simulink model "debugIMU"  (Simulink 9.0)
settings: Solver=FixedStepDiscrete  StartTime=0.0  StopTime=inf  FixedStep=0.01  RelTol=1e-3  EnableMultiTasking=on
InitFcn:
  | ROBOT_DOF=23;
libraries: WBToolboxLibrary x6
settings Model: SuppressorTable=22 serialization::archive 11 0 6 0 0 0 11 0  Creator=DanielePucci  LastModifiedBy=icub
settings DataIOCC: LimitDataPoints=on  SaveFormat=StructureWithTime
settings DebuggingCC: UnderspecifiedInitializationDetection=Simplified  MergeDetectMultiDrivingBlocksExec=error
settings HardwareCC: ProdBitPerPointer=64  ProdLargestAtomicFloat=Float  ProdIntDivRoundTo=Zero  ProdEndianess=LittleEndian  ProdHWDeviceType=Specified

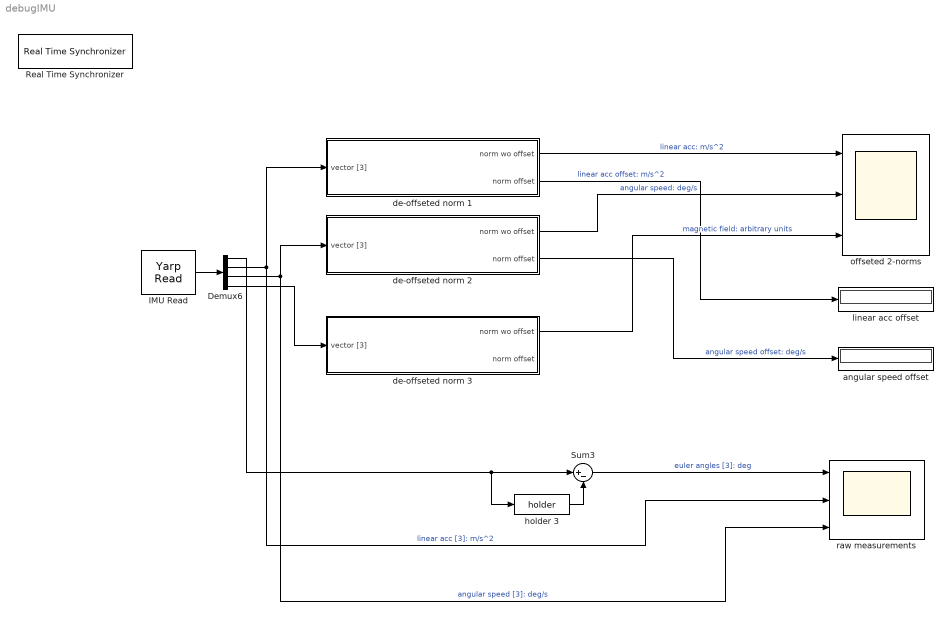
== system debugIMU ==
  Demux6 : Demux
  IMU Read : WBToolboxLibrary/Utilities/Yarp Read  portName='/icub/inertial'  signalSize=12  blocking=off  timestamp=off  autoconnect=on  errorOnConnection=off
      settings: SourceProductName=Whole Body Toolbox
  Real Time Synchronizer : WBToolboxLibrary/Utilities/Real Time Synchronizer  period=0.01
      settings: SourceProductName=Whole Body Toolbox
  Sum3 : Sum  Inputs=|+-
  angular speed offset : Display
  de-offseted norm 1 : Subsystem
  de-offseted norm 2 : Subsystem
  de-offseted norm 3 : Subsystem
  holder 3 : WBToolboxLibrary/Utilities/holder 
      settings: SourceProductName=Whole Body Toolbox
  linear acc offset : Display
  offseted 2-norms : Scope  NumInputPorts=3
  raw measurements : Scope  NumInputPorts=3
  wires:
  IMU Read/1 -> Demux6/1
  de-offseted norm 2/2(norm offset) -> angular speed offset/1  "angular speed offset: deg/s"
  de-offseted norm 2/1(norm wo offset) -> offseted 2-norms/2  "angular speed: deg/s"
  de-offseted norm 3/1(norm wo offset) -> offseted 2-norms/3  "magnetic field: arbitrary units"
  Demux6/2 -> de-offseted norm 1/1(vector [3]), raw measurements/2  "linear acc [3]: m/s^2"
  Demux6/3 -> de-offseted norm 2/1(vector [3]), raw measurements/3  "angular speed [3]: deg/s"
  Demux6/4 -> de-offseted norm 3/1(vector [3])
  Sum3/1 -> raw measurements/1  "euler angles [3]: deg"
  Demux6/1 -> holder 3/1, Sum3/1
  holder 3/1 -> Sum3/2
  de-offseted norm 1/1(norm wo offset) -> offseted 2-norms/1  "linear acc: m/s^2"
  de-offseted norm 1/2(norm offset) -> linear acc offset/1  "linear acc offset: m/s^2"

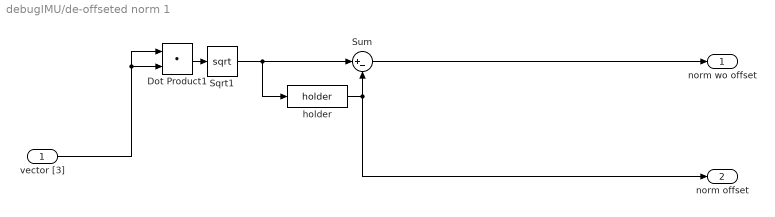
== system debugIMU/de-offseted norm 1 ==
  vector [3] : Inport
  Dot Product1 : DotProduct  InputSameDT=on  OutDataTypeStr=Inherit: Inherit via internal rule
  Sqrt1 : Sqrt  SaturateOnIntegerOverflow=on
  Sum : Sum  Inputs=|+-
  "holder " : WBToolboxLibrary/Utilities/holder 
      settings: SourceProductName=Whole Body Toolbox
  norm wo offset : Outport
  norm offset : Outport  Port=2
  wires:
  "holder "/1 -> norm offset/1, Sum/2
  Sqrt1/1 -> "holder "/1, Sum/1
  Sum/1 -> norm wo offset/1
  Dot Product1/1 -> Sqrt1/1
  vector [3]/1 -> Dot Product1/1, Dot Product1/2

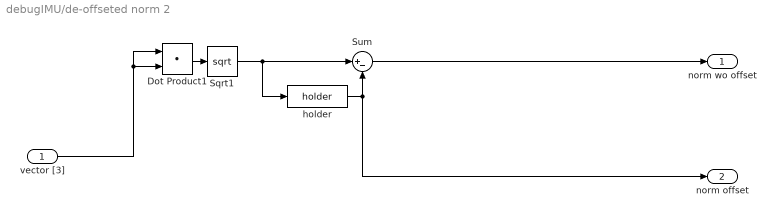
== system debugIMU/de-offseted norm 2 ==
  vector [3] : Inport
  Dot Product1 : DotProduct  InputSameDT=on  OutDataTypeStr=Inherit: Inherit via internal rule
  Sqrt1 : Sqrt  SaturateOnIntegerOverflow=on
  Sum : Sum  Inputs=|+-
  "holder " : WBToolboxLibrary/Utilities/holder 
      settings: SourceProductName=Whole Body Toolbox
  norm wo offset : Outport
  norm offset : Outport  Port=2
  wires:
  "holder "/1 -> norm offset/1, Sum/2
  Sqrt1/1 -> "holder "/1, Sum/1
  Sum/1 -> norm wo offset/1
  Dot Product1/1 -> Sqrt1/1
  vector [3]/1 -> Dot Product1/1, Dot Product1/2

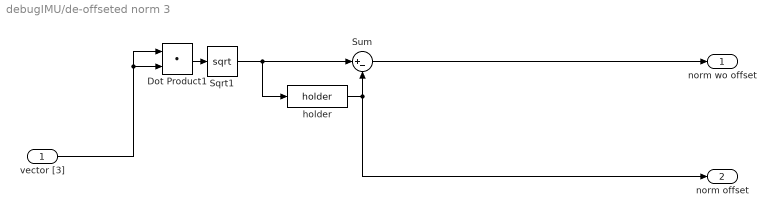
== system debugIMU/de-offseted norm 3 ==
  vector [3] : Inport
  Dot Product1 : DotProduct  InputSameDT=on  OutDataTypeStr=Inherit: Inherit via internal rule
  Sqrt1 : Sqrt  SaturateOnIntegerOverflow=on
  Sum : Sum  Inputs=|+-
  "holder " : WBToolboxLibrary/Utilities/holder 
      settings: SourceProductName=Whole Body Toolbox
  norm wo offset : Outport
  norm offset : Outport  Port=2
  wires:
  "holder "/1 -> norm offset/1, Sum/2
  Sqrt1/1 -> "holder "/1, Sum/1
  Sum/1 -> norm wo offset/1
  Dot Product1/1 -> Sqrt1/1
  vector [3]/1 -> Dot Product1/1, Dot Product1/2
